simulink model "ballbeam_sim"  (R2016b)
settings: Solver=ode45  StartTime=0.0  StopTime=P.t_end  RelTol=1e-3  EnableMultiTasking=on
InitFcn:
  | addpath ./..
  | ballbeam_param
  | ballbeamParamHWf
undefined symbols (not defined in the file or in its folder): ballbeam_animation, P
settings Model: Creator=beard  LastModifiedBy=mclain
settings DataIOCC: LimitDataPoints=on  SaveFormat=Array  SignalLoggingSaveFormat=ModelDataLogs
settings OptimizationCC: ExpressionDepthLimit=2147483647  InitFltsAndDblsToZero=on  LifeSpan=inf
settings DebuggingCC: UnderspecifiedInitializationDetection=Classic  MergeDetectMultiDrivingBlocksExec=none  SolverPrmCheckMsg=warning  FcnCallInpInsideContextMsg=warning  StateNameClashWarn=warning  SFUnexpectedBacktrackingDiag=warning  SFNoUnconditionalDefaultTransitionDiag=warning  SFExecutionAtInitializationDiag=none
settings HardwareCC: ProdBitPerPointer=32  ProdBitPerSizeT=32  ProdBitPerPtrDiffT=32  ProdLargestAtomicFloat=None  ProdIntDivRoundTo=Undefined  ProdEndianess=Unspecified  ProdWordSize=32  ProdHWDeviceType=32-bit Generic
settings ModelReferenceCC: PropagateSignalLabelsOutOfModel=off
settings GRTTargetCC: TargetLangStandard=C89/C90 (ANSI)  GeneratePreprocessorConditionals=Disable all  CombineOutputUpdateFcns=off  GRTInterface=on
settings ConfigComp: CovMetricSettings=dw  CovHtmlReporting=on  CovSaveCumulativeToWorkspaceVar=on  CovSaveSingleToWorkspaceVar=on  CovExternalEMLEnable=off

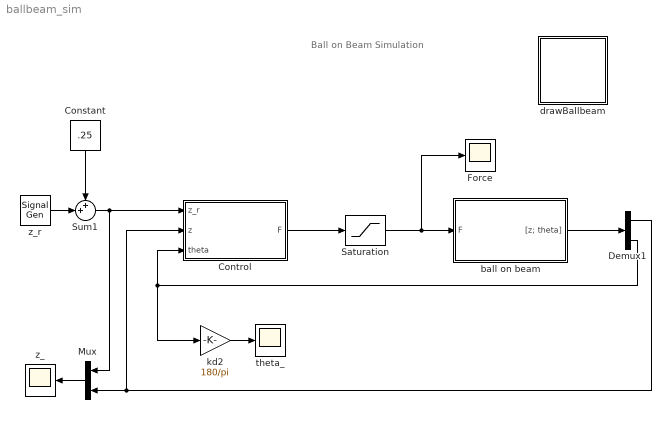
== system ballbeam_sim ==
  note: Ball on Beam Simulation
  Constant : Constant  Value=.25
  Control : Subsystem
  Demux1 : Demux  Outputs=2
  Force : Scope
  Mux : Mux  Inputs=2
  Saturation : Saturate  UpperLimit=P.Fmax  LowerLimit=-P.Fmax
  Sum1 : Sum  Inputs=++|
  ball on beam : Subsystem
  drawBallbeam : Subsystem
      mask Display: image(imread('tv.jpg'))
  kd2 : Gain  Gain=180/pi
  theta_ : Scope
  z_ : Scope
  z_r : SignalGenerator  WaveForm=square  Amplitude=0.125  Frequency=.02
  wires:
  z_r/1 -> Sum1/2
  Constant/1 -> Sum1/1
  Control/1(F) -> Saturation/1
  ball on beam/1("[z; theta]") -> Demux1/1
  Demux1/2 -> kd2/1, Control/3(theta)
  Demux1/1 -> Control/2(z), Mux/2
  Mux/1 -> z_/1
  kd2/1 -> theta_/1
  Sum1/1 -> Mux/1, Control/1(z_r)
  Saturation/1 -> ball on beam/1(F), Force/1

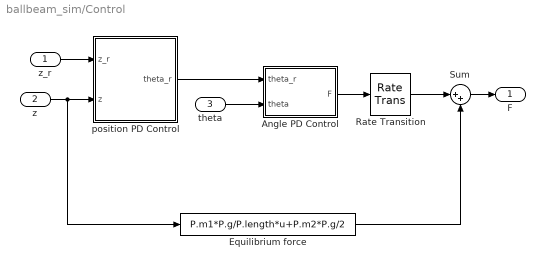
== system ballbeam_sim/Control ==
  z_r : Inport
  z : Inport  Port=2
  theta : Inport  Port=3
  "Angle PD Control " : Subsystem
  Equilibrium force : Fcn  Expr=P.m1*P.g/P.length*u+P.m2*P.g/2
  Rate Transition : RateTransition  OutPortSampleTime=P.Ts
  Sum : Sum  Inputs=|++
  position PD Control : Subsystem
  F : Outport
  wires:
  theta/1 -> "Angle PD Control "/2(theta)
  z_r/1 -> position PD Control/1(z_r)
  position PD Control/1(theta_r) -> "Angle PD Control "/1(theta_r)
  "Angle PD Control "/1(F) -> Rate Transition/1
  Sum/1 -> F/1
  z/1 -> Equilibrium force/1, position PD Control/2(z)
  Rate Transition/1 -> Sum/1
  Equilibrium force/1 -> Sum/2

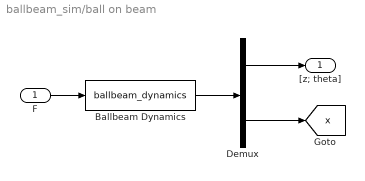
== system ballbeam_sim/ball on beam ==
  F : Inport
  Ballbeam Dynamics : S-Function  FunctionName=ballbeam_dynamics  Parameters=P  SFunctionDeploymentMode=off  EnableBusSupport=off
  Demux : Demux  Outputs=[2;4]
  "[z; theta]" : Outport
  tag scope: x=global
  wires:
  Demux/2 -> [x]
  Demux/1 -> "[z; theta]"/1
  Ballbeam Dynamics/1 -> Demux/1
  F/1 -> Ballbeam Dynamics/1

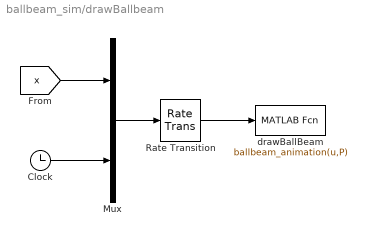
== system ballbeam_sim/drawBallbeam ==
  Clock : Clock
  Mux : Mux  Inputs=2
  Rate Transition : RateTransition  OutPortSampleTime=P.t_plot
  drawBallBeam : MATLABFcn  MATLABFcn=ballbeam_animation(u,P)  OutputDimensions=0
  wires:
  Mux/1 -> Rate Transition/1
  [x] -> Mux/1
  Clock/1 -> Mux/2
  Rate Transition/1 -> drawBallBeam/1

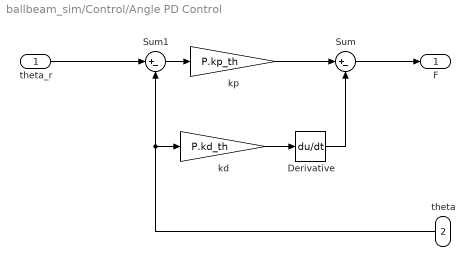
== system ballbeam_sim/Control/Angle PD Control  ==
  theta_r : Inport
  theta : Inport  Port=2
  Derivative : Derivative  CoefficientInTFapproximation=P.sigma
  Sum : Sum  Inputs=|+-
  Sum1 : Sum  Inputs=|+-
  kd : Gain  Gain=P.kd_th
  kp : Gain  Gain=P.kp_th
  F : Outport
  wires:
  theta_r/1 -> Sum1/1
  Sum/1 -> F/1
  theta/1 -> kd/1, Sum1/2
  Sum1/1 -> kp/1
  kp/1 -> Sum/1
  kd/1 -> Derivative/1
  Derivative/1 -> Sum/2

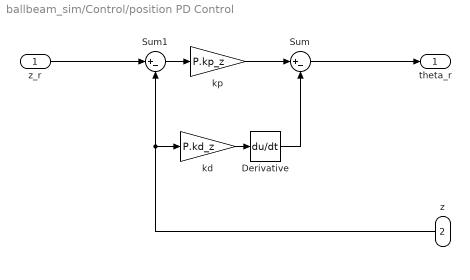
== system ballbeam_sim/Control/position PD Control ==
  z_r : Inport
  z : Inport  Port=2
  Derivative : Derivative  CoefficientInTFapproximation=P.sigma
  Sum : Sum  Inputs=|+-
  Sum1 : Sum  Inputs=|+-
  kd : Gain  Gain=P.kd_z
  kp : Gain  Gain=P.kp_z
  theta_r : Outport
  wires:
  z_r/1 -> Sum1/1
  Sum/1 -> theta_r/1
  z/1 -> kd/1, Sum1/2
  Sum1/1 -> kp/1
  kp/1 -> Sum/1
  kd/1 -> Derivative/1
  Derivative/1 -> Sum/2
